simulink library "MicDiag"  (R2022b)
settings: Solver=VariableStepAuto  StartTime=0.0  StopTime=10.0  RelTol=1e-3
values from neighbouring files (symbols this model uses):
  numMicIn = 2    [PhaseDetector_init.m]
undefined symbols (not defined in the file or in its folder): framesize
libraries: MicDiagBtc x1
settings Model: Creator=pk47312  LastModifiedBy=kl13806
settings SolverCC: AlgebraicLoopSolver=TrustRegion
settings DebuggingCC: UnconnectedInputMsg=warning  UnconnectedOutputMsg=warning  UnconnectedLineMsg=warning  SFMachineParentedDataDiag=warning
settings ModelReferenceCC: EnableRefExpFcnMdlSchedulingChecks=on
settings RTWCC: DLArmComputeVersion=19.05

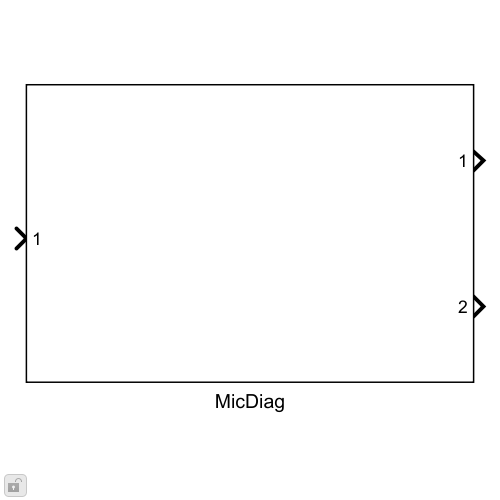
[thumbnail: Simulink's stored preview of the top-level diagram]
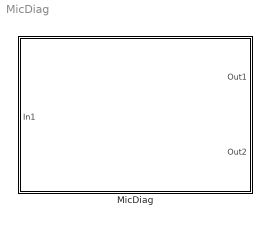
== system MicDiag ==
  MicDiag : Subsystem  mask{numMicIn=numMicIn, framesize=framesize}
      mask prompts: numMicIn "number of Microphone"; framesize "Frame Size"
      mask help: MicDiag accumulates the sum of squares for multiple channels individually
      mask init:
      | blkh = gcbh;
      | % Copy discrete mask parameters into a classdef object
      | InnerLinkConfig = MicDiagConfig;
      | InnerLinkConfig.NumMicIn = numMicIn;
      | InnerLinkConfig.FrameSize = framesize;

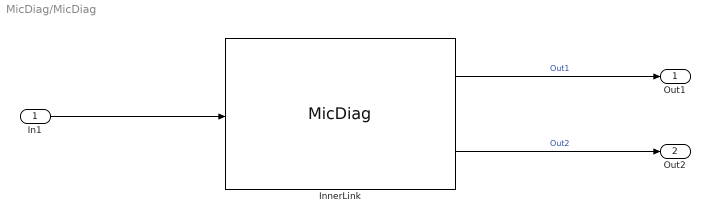
== system MicDiag/MicDiag ==
  In1 : Inport
  InnerLink : MicDiagBtc/MicDiag  Config=InnerLinkConfig  FeatureName=MicDiag
      settings: SourceProductName=Bose Blocklib
  Out1 : Outport
  Out2 : Outport  Port=2
  wires:
  InnerLink/1 -> Out1/1  "Out1"
  InnerLink/2 -> Out2/1  "Out2"
  In1/1 -> InnerLink/1
